simulink model "simulink_MotorDC"  (R2022b)
settings: Solver=VariableStepAuto  StartTime=0.0  StopTime=10.0  RelTol=1e-3
values from neighbouring files (symbols this model uses):
  A = [-R/L -ke/L ... (first row only)    [MotorDC.m]
  B = [1/L 0 ... (first row only)    [MotorDC.m]
  C = [1 0 ... (first row only)    [MotorDC.m]
  D = zeros(rows_C, columns_B)    [MotorDC.m]
settings Model: Creator=elisa  LastModifiedBy=elisa

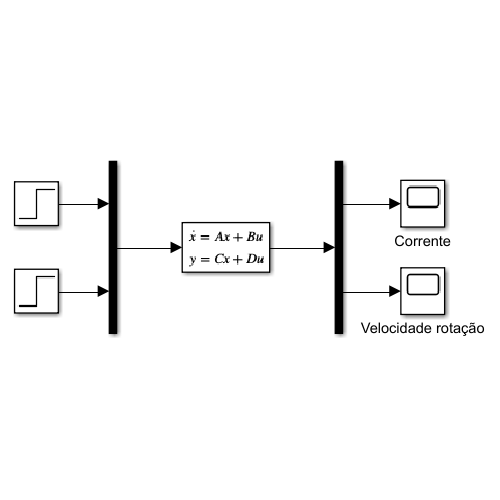
[thumbnail: Simulink's stored preview of the top-level diagram]
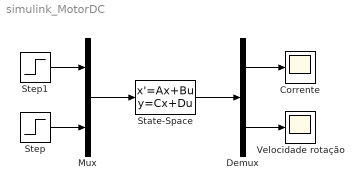
== system simulink_MotorDC ==
  Corrente : Scope
  Demux : Demux  Outputs=2
  Mux : Mux  Inputs=2
  State-Space : StateSpace  A=A  B=B  C=C  D=D  InitialCondition=0  ParameterTunability=Optimized
  Step : Step  Time=10  After=0.091  SampleTime=20
  Step1 : Step  Time=20  Before=10  After=10  SampleTime=20
  Velocidade rotação : Scope
  wires:
  Mux/1 -> State-Space/1
  Step/1 -> Mux/2
  Step1/1 -> Mux/1
  State-Space/1 -> Demux/1
  Demux/1 -> Corrente/1
  Demux/2 -> Velocidade rotação/1
